simulink model "sampleModel1663"  (R2023a)
settings: Solver=VariableStepAuto  StartTime=0.0  StopTime=10.0  RelTol=1e-3
libraries: hdlsllib x8, simulink x1
settings Model: Creator=user1  LastModifiedBy=user1

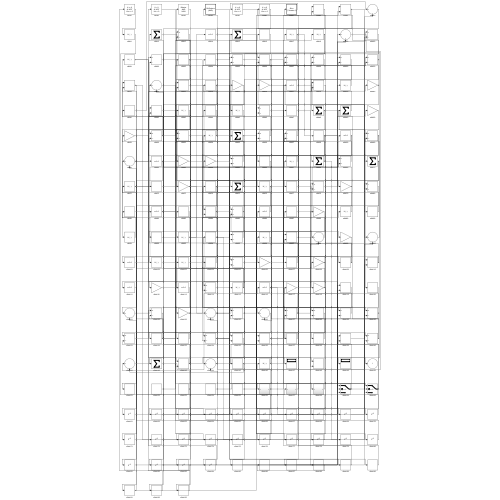
[thumbnail: Simulink's stored preview of the top-level diagram]
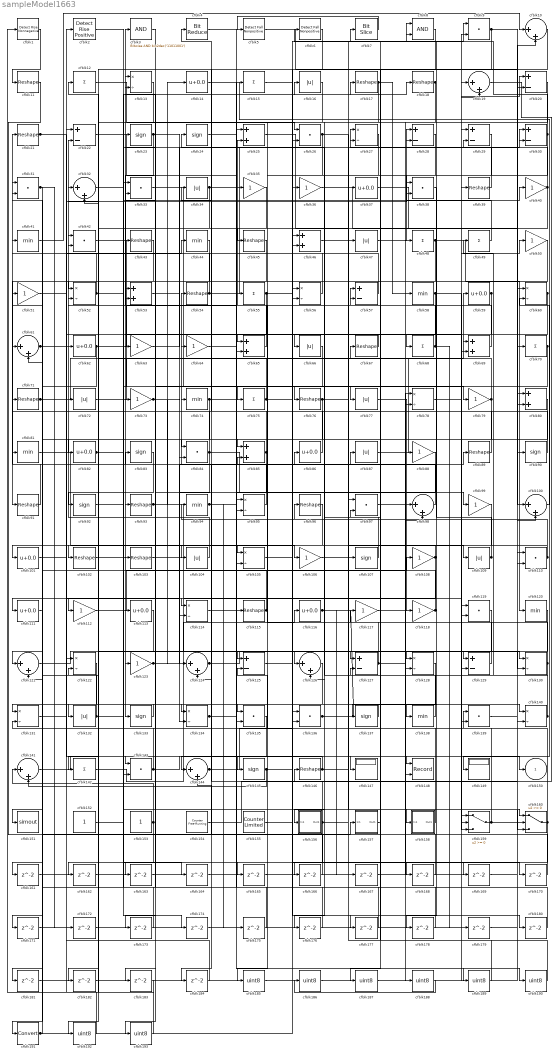
== system sampleModel1663 ==
  cfblk1 : hdlsllib/Logic and Bit Operations/Detect Rise Nonnegative  vinit=0  OutDataTypeStr=boolean
  cfblk{10,19,32,61,98,100,121,124,126,141,144} (11 alike) : Sum  Inputs=|++
  cfblk{14,37,59,62,82,86,101,111,113,116} (10 alike) : Bias  Bias=0.0  SaturateOnIntegerOverflow=off
  cfblk{11,17..18,21,39,43,45,54,67,71,76,89,91,93,96,102..103,115,146} (19 alike) : Reshape
  cfblk{16,34,47,66,72,77,87,104,109,132} (10 alike) : Abs  SaturateOnIntegerOverflow=off
  cfblk{13,27,52,56,60,78,95,105,114,122,128,130..131,134,140} (15 alike) : Product  Inputs=*/  RndMeth=Zero  SaturateOnIntegerOverflow=on
  cfblk{35..36,40,50..51,63..64,73,79,88,99,106,108,112,117..118,123} (17 alike) : Gain
  cfblk{23..24,83,90,92,107,133,137,145} (9 alike) : Signum
  cfblk{9,26,31,33,38,42,84,97,110,119,135..136,139,143} (14 alike) : DotProduct  OutDataTypeStr=Inherit: Inherit via internal rule
  cfblk{12,15,48..49,55,68,70,75,142} (9 alike) : Sum  Inputs=+
  cfblk{41,44,58,74,81,94,120,138} (8 alike) : MinMax
  cfblk{20,22,28..30,57,125,127,129} (9 alike) : Sum  Inputs=+-
  cfblk147 : Display
  cfblk148 : Record  FileSettingsInternal="{\"entries\":[{\"content\":{\"excelSettings\":{\"content\":{},\"type\":\"Streamout.ExcelSettings\"}},\"type\":\"Streamout.FileSettingStorage\",\"uuid\":\"\"}],\"packageUris\":[\"http:\\/\\/schema.mathworks.com\\/mf0\\/streamout_blocks\\/R2020a\"],\"version\":\"1.0\"}"  Layout=[1 1]  SignalsInternal="{\"entries\":[{\"content\":{\"signals\":[{\"content\":{\"blockPath\":[],\"dimensions\":[1],\"domain\":\"\",\"lineColor\":\"#a2142f\",\"plots\":[1],\"port\":1,\"signalID\":2664,\"signalName\":\"XY Graph:1\"},\"type\":\"RecordBlkView.Signal\",\"uuid\":\"\"},{\"content\":{\"blockPath\":[],\"dimensions\":[1],\"domain\":\"\",\"lineColor\":\"#139fff\",\"plots\":[1],\"port\":2,\"signalID\":2667,\"signalName\":\"XY Graph:2\"},\"type\":\"RecordBlkView.Signal\",\"uuid\":\"\"}]},\"type\":\"RecordBlkView.InputSignals\",\"uuid\":\"\"}],\"packageUris\":[\"http:\\/\\/schema.mathworks.com\\/mf0\\/streamout_blocks\\/R2020a\"],\"version\":\"1.0\"}"  VisualizationBindings="{\"xyplotplugin\":{\"info\":[{\"series\":[{\"bindingParametersList\":[{\"parameter\":\"X-Axis\",\"signalID\":2664,\"signalName\":\"XY Graph:1\"},{\"parameter\":\"Y-Axis\",\"signalID\":2667,\"signalName\":\"XY Graph:2\"}],\"seriesID\":8670}],\"subplotID\":1}]}}"  CompatibilityTag=XY  st=-1
  cfblk149 : Display
  cfblk151 : ToWorkspace  VariableName=simout  SaveFormat=Timeseries  SampleTime=-1
  cfblk152 : Constant  SampleTime=-1
  cfblk153 : Constant  SampleTime=-1
  cfblk154 : hdlsllib/Sources/Counter Free-Running  NumBits=16  tsamp=-1
  cfblk155 : hdlsllib/Sources/Counter Limited  uplimit=7  tsamp=-1
  cfblk156 : Subsystem
      settings: LibrarySourceBlock=|
      | hdlsllib/Ports &
      | Subsystems/Subsystem
  cfblk157 : Subsystem
      settings: LibrarySourceBlock=|
      | hdlsllib/Ports &
      | Subsystems/Subsystem
  cfblk158 : Subsystem
      settings: LibrarySourceBlock=|
      | hdlsllib/Ports &
      | Subsystems/Subsystem
  cfblk159 : Switch  SaturateOnIntegerOverflow=off  InputSameDT=off
  cfblk160 : Switch  SaturateOnIntegerOverflow=off  InputSameDT=off
  cfblk{161..184} (24 alike) : Delay  SampleTime=1
  cfblk{185..190,192..193} (8 alike) : DataTypeConversion  OutDataTypeStr=uint8  SaturateOnIntegerOverflow=off  RndMeth=Floor
  cfblk191 : DataTypeConversion  SaturateOnIntegerOverflow=off  RndMeth=Floor
  cfblk2 : hdlsllib/Logic and Bit Operations/Detect Rise Positive  vinit=0  OutDataTypeStr=boolean
  cfblk{25,46,53,65,69,80,85} (7 alike) : Sum
  cfblk3 : simulink/Logic and Bit Operations/Bitwise Operator  logicop=AND  UseBitMask=on  BitMask=bin2dec('11011001')  BitMaskRealWorld=Stored Integer
      settings: LibrarySourceBlock=|
      | hdlsllib/Logic and Bit
      | Operations/Bitwise
      | Operator
  cfblk4 : hdlsllib/Logic and Bit Operations/Bit Reduce  mode=AND
  cfblk5 : hdlsllib/Logic and Bit Operations/Detect Fall Nonpositive  vinit=0  OutDataTypeStr=boolean
  cfblk6 : hdlsllib/Logic and Bit Operations/Detect Fall Nonpositive  vinit=0  OutDataTypeStr=boolean
  cfblk7 : hdlsllib/Logic and Bit Operations/Bit Slice  lidx=7  ridx=0
  cfblk8 : Logic  AllPortsSameDT=off  OutDataTypeStr=boolean
  cfblk150 : Outport  VectorParamsAs1DForOutWhenUnconnected=off
  wires:
  cfblk91/1 -> cfblk21/1
  cfblk23/1 -> cfblk133/1, cfblk125/1
  cfblk45/1 -> cfblk91/1
  cfblk67/1 -> cfblk66/1
  cfblk109/1 -> cfblk96/1, cfblk8/2
  cfblk55/1 -> cfblk134/2, cfblk177/1
  cfblk28/1 -> cfblk77/1
  cfblk88/1 -> cfblk105/1
  cfblk14/1 -> cfblk149/1
  cfblk77/1 -> cfblk118/1
  cfblk75/1 -> cfblk12/1, cfblk180/1
  cfblk129/1 -> cfblk57/1
  cfblk69/1 -> cfblk3/1
  cfblk34/1 -> cfblk93/1, cfblk159/2
  cfblk58/1 -> cfblk68/1, cfblk50/1, cfblk160/3, cfblk63/1
  cfblk54/1 -> cfblk19/1, cfblk42/1
  cfblk87/1 -> cfblk59/1
  cfblk19/1 -> cfblk146/1
  cfblk33/1 -> cfblk79/1
  cfblk17/1 -> cfblk126/1, cfblk58/1
  cfblk59/1 -> cfblk128/1, cfblk159/3
  cfblk141/1 -> cfblk143/1
  cfblk142/1 -> cfblk116/1
  cfblk79/1 -> cfblk126/2, cfblk32/1
  cfblk48/1 -> cfblk120/1, cfblk84/2
  cfblk94/1 -> cfblk89/1, cfblk175/1
  cfblk99/1 -> cfblk156/1(In1)
  cfblk81/1 -> cfblk106/1
  cfblk93/1 -> cfblk130/1, cfblk14/1
  cfblk159/1 -> cfblk80/1, cfblk27/2
  cfblk86/1 -> cfblk54/1
  cfblk18/1 -> cfblk134/1, cfblk148/2
  cfblk113/1 -> cfblk143/2
  cfblk65/1 -> cfblk25/2
  cfblk24/1 -> cfblk16/1
  cfblk146/1 -> cfblk47/1, cfblk145/1
  cfblk78/1 -> cfblk20/1
  cfblk12/1 -> cfblk26/1
  cfblk11/1 -> cfblk157/1(In1)
  cfblk50/1 -> cfblk101/1
  cfblk135/1 -> cfblk144/1
  cfblk7/1 -> cfblk5/1
  cfblk104/1 -> cfblk22/2
  cfblk36/1 -> cfblk90/1
  cfblk107/1 -> cfblk86/1
  cfblk136/1 -> cfblk140/1, cfblk18/1
  cfblk5/1 -> cfblk100/1
  cfblk121/1 -> cfblk123/1
  cfblk130/1 -> cfblk55/1, cfblk127/2
  cfblk110/1 -> cfblk94/1, cfblk103/1
  cfblk70/1 -> cfblk114/1, cfblk168/1
  cfblk85/1 -> cfblk34/1, cfblk105/2
  cfblk153/1 -> cfblk141/1, cfblk192/1
  cfblk134/1 -> cfblk147/1, cfblk38/2, cfblk190/1
  cfblk112/1 -> cfblk108/1
  cfblk72/1 -> cfblk69/1
  cfblk139/1 -> cfblk110/1
  cfblk42/1 -> cfblk75/1
  cfblk101/1 -> cfblk2/1
  cfblk157/1(Out1) -> cfblk7/1
  cfblk44/1 -> cfblk73/1
  cfblk20/1 -> cfblk45/1
  cfblk156/1(Out1) -> cfblk83/1, cfblk8/1, cfblk193/1
  cfblk41/1 -> cfblk10/1
  cfblk82/1 -> cfblk128/2, cfblk40/1
  cfblk31/1 -> cfblk171/1, cfblk172/1
  cfblk108/1 -> cfblk111/1, cfblk104/1
  cfblk21/1 -> cfblk62/1, cfblk69/2
  cfblk118/1 -> cfblk81/1, cfblk138/1
  cfblk132/1 -> cfblk51/1, cfblk28/2, cfblk164/1
  cfblk116/1 -> cfblk137/1, cfblk167/1
  cfblk152/1 -> cfblk43/1
  cfblk95/1 -> cfblk74/1
  cfblk43/1 -> cfblk102/1
  cfblk25/1 -> cfblk107/1
  cfblk100/1 -> cfblk60/2
  cfblk89/1 -> cfblk33/2
  cfblk137/1 -> cfblk132/1
  cfblk84/1 -> cfblk61/1, cfblk98/1, cfblk183/1
  cfblk92/1 -> cfblk158/1(In1)
  cfblk155/1 -> cfblk9/1
  cfblk13/1 -> cfblk82/1
  cfblk47/1 -> cfblk78/2
  cfblk52/1 -> cfblk31/1, cfblk17/1
  cfblk16/1 -> cfblk52/1
  cfblk49/1 -> cfblk28/1
  cfblk90/1 -> cfblk64/1
  cfblk74/1 -> cfblk99/1, cfblk84/1
  cfblk26/1 -> cfblk135/1, cfblk130/2
  cfblk53/1 -> cfblk129/1
  cfblk124/1 -> cfblk127/1, cfblk67/1
  cfblk76/1 -> cfblk160/2, cfblk181/1
  cfblk73/1 -> cfblk95/2, cfblk124/1
  cfblk102/1 -> cfblk113/1
  cfblk35/1 -> cfblk53/1
  cfblk127/1 -> cfblk117/1, cfblk98/2
  cfblk2/1 -> cfblk76/1
  cfblk158/1(Out1) -> cfblk61/2
  cfblk64/1 -> cfblk15/1
  cfblk144/1 -> cfblk36/1, cfblk124/2
  cfblk106/1 -> cfblk37/1
  cfblk98/1 -> cfblk31/2
  cfblk122/1 -> cfblk191/1
  cfblk145/1 -> cfblk141/2, cfblk30/2
  cfblk30/1 -> cfblk48/1, cfblk6/1
  cfblk22/1 -> cfblk115/1
  cfblk103/1 -> cfblk159/1
  cfblk40/1 -> cfblk29/2, cfblk92/1
  cfblk138/1 -> cfblk87/1
  cfblk4/1 -> cfblk160/1
  cfblk29/1 -> cfblk46/2
  cfblk125/1 -> cfblk26/2
  cfblk39/1 -> cfblk27/1
  cfblk57/1 -> cfblk41/1
  cfblk96/1 -> cfblk121/1
  cfblk60/1 -> cfblk65/1, cfblk85/1
  cfblk46/1 -> cfblk109/1
  cfblk71/1 -> cfblk9/2, cfblk114/2
  cfblk10/1 -> cfblk112/1
  cfblk1/1 -> cfblk11/1
  cfblk140/1 -> cfblk24/1, cfblk49/1
  cfblk68/1 -> cfblk42/2, cfblk179/1
  cfblk115/1 -> cfblk13/1, cfblk52/2
  cfblk37/1 -> cfblk80/2
  cfblk131/1 -> cfblk44/1
  cfblk123/1 -> cfblk23/1, cfblk85/2
  cfblk61/1 -> cfblk38/1, cfblk150/1
  cfblk117/1 -> cfblk88/1
  cfblk63/1 -> cfblk30/1
  cfblk62/1 -> cfblk35/1, cfblk151/1
  cfblk9/1 -> cfblk70/1, cfblk56/2
  cfblk143/1 -> cfblk53/2, cfblk148/1, cfblk32/2
  cfblk154/1 -> cfblk100/2
  cfblk83/1 -> cfblk142/1
  cfblk160/1 -> cfblk139/1, cfblk125/2, cfblk176/1
  cfblk56/1 -> cfblk4/1
  cfblk133/1 -> cfblk131/1
  cfblk126/1 -> cfblk135/2
  cfblk51/1 -> cfblk72/1
  cfblk111/1 -> cfblk161/1
  cfblk161/1 -> cfblk19/2
  cfblk128/1 -> cfblk162/1
  cfblk162/1 -> cfblk78/1
  cfblk3/1 -> cfblk163/1
  cfblk163/1 -> cfblk25/1
  cfblk164/1 -> cfblk65/2
  cfblk80/1 -> cfblk165/1
  cfblk165/1 -> cfblk60/1
  cfblk27/1 -> cfblk166/1
  cfblk166/1 -> cfblk46/1
  cfblk167/1 -> cfblk129/2
  cfblk168/1 -> cfblk131/2
  cfblk15/1 -> cfblk169/1
  cfblk169/1 -> cfblk10/2
  cfblk105/1 -> cfblk170/1
  cfblk170/1 -> cfblk144/2
  cfblk171/1 -> cfblk110/2
  cfblk172/1 -> cfblk139/2
  cfblk66/1 -> cfblk173/1
  cfblk173/1 -> cfblk33/1
  cfblk32/1 -> cfblk174/1
  cfblk174/1 -> cfblk56/1
  cfblk175/1 -> cfblk121/2
  cfblk176/1 -> cfblk13/2
  cfblk177/1 -> cfblk95/1
  cfblk38/1 -> cfblk178/1
  cfblk178/1 -> cfblk57/2
  cfblk179/1 -> cfblk20/2
  cfblk180/1 -> cfblk136/1
  cfblk181/1 -> cfblk140/2
  cfblk120/1 -> cfblk182/1
  cfblk182/1 -> cfblk29/1
  cfblk183/1 -> cfblk1/1
  cfblk6/1 -> cfblk184/1
  cfblk184/1 -> cfblk22/1
  cfblk119/1 -> cfblk185/1
  cfblk185/1 -> cfblk39/1
  cfblk186/1 -> cfblk119/1
  cfblk8/1 -> cfblk187/1
  cfblk187/1 -> cfblk119/2
  cfblk97/1 -> cfblk188/1
  cfblk188/1 -> cfblk186/1
  cfblk114/1 -> cfblk189/1
  cfblk189/1 -> cfblk97/1
  cfblk190/1 -> cfblk97/2
  cfblk191/1 -> cfblk136/2, cfblk71/1
  cfblk192/1 -> cfblk122/1
  cfblk193/1 -> cfblk122/2

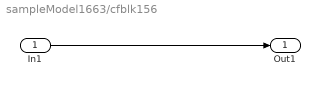
== system sampleModel1663/cfblk156 ==
  In1 : Inport
  Out1 : Outport
  wires:
  In1/1 -> Out1/1

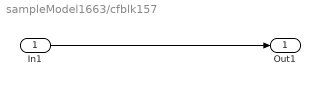
== system sampleModel1663/cfblk157 ==
  In1 : Inport
  Out1 : Outport
  wires:
  In1/1 -> Out1/1

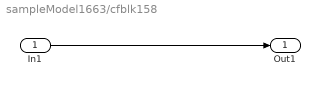
== system sampleModel1663/cfblk158 ==
  In1 : Inport
  Out1 : Outport
  wires:
  In1/1 -> Out1/1
